simulink model "EV_motor_model"  (R2023a)
settings: Solver=ode15s  StartTime=0.0  StopTime=200  RelTol=1e-3
values from neighbouring files (symbols this model uses):
  A = 1.8    [evmodel.m]    (also in params.mat)
  B = 2e-4    (= 0.0002)    [evmodel.m]    (also in params.mat)
  Cd = 0.3    [evmodel.m]    (also in params.mat)
  G = 11    [params.mat]
  J = 0.05    [evmodel.m]    (also in params.mat)
  La = 0.003004    [params.mat]
  Laf = 0.001766    [evmodel.m]    (also in params.mat)
  Lf = 0.003004    [params.mat]
  m = 800    [evmodel.m]    (also in params.mat)
  mu_rr = 0.015    [params.mat]
  r = 0.25    [evmodel.m]    (also in params.mat = 0.3)
  Ra = 0.06    [params.mat]
  Rf = 0.06    [params.mat]
  rho = 1.25    [evmodel.m]    (also in params.mat)
undefined symbols (not defined in the file or in its folder): DiscIntNeverNeededParam
libraries: slpidlib x5, eePwmGenerator x1, spsTriangleGeneratorLib x1
settings Model: Creator=HP  LastModifiedBy=karti
settings DebuggingCC: AlgebraicLoopMsg=none  UnconnectedInputMsg=warning  UnconnectedOutputMsg=warning  UnconnectedLineMsg=warning
settings ModelReferenceCC: EnableRefExpFcnMdlSchedulingChecks=on
settings RTWCC: DLArmComputeVersion=19.05

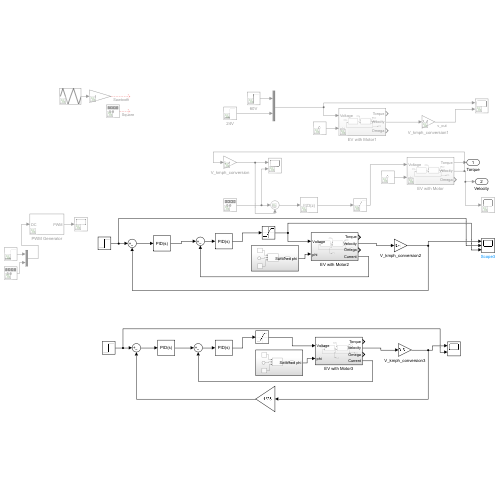
[thumbnail: Simulink's stored preview of the top-level diagram]
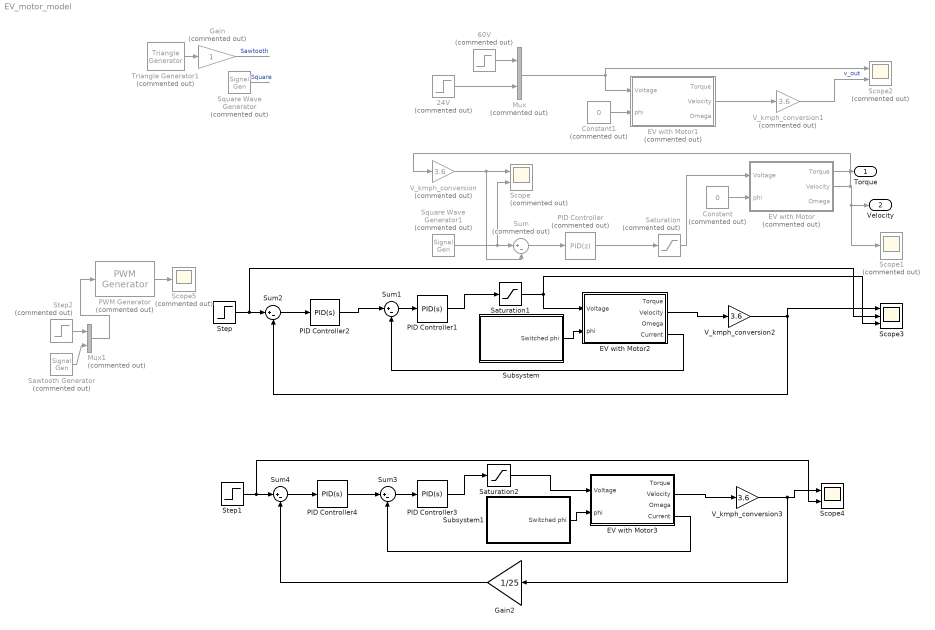
== system EV_motor_model ==
  24V : Step  Commented=on  Time=0  After=24  SampleTime=0
  60V : Step  Commented=on  Time=0  After=60  SampleTime=0
  Constant : Constant  Commented=on  Value=0
  Constant1 : Constant  Commented=on  Value=0
  EV with Motor : Subsystem  Commented=on
  EV with Motor1 : Subsystem  Commented=on
  EV with Motor2 : Subsystem
  EV with Motor3 : Subsystem
  Gain : Gain  Commented=on
  Gain2 : Gain  Gain=1/25
  Mux : Mux  Commented=on  Inputs=2
  Mux1 : Mux  Commented=on  Inputs=2
  PID Controller : slpidlib/PID Controller  Commented=on  Controller=PID  Form=Parallel  TimeDomain=Discrete-time  UseExternalTs=off  SampleTime=-1  IntegratorMethod=Forward Euler  FilterMethod=Forward Euler  ControllerParametersSource=internal  P=21.8052  I=4.7645  UseKiTs=off  D=2  N=100  UseFilter=on  TunerSelectOption=Frequency Response Based  InitialConditionSource=internal  InitialConditionForIntegrator=0  InitialConditionForFilter=0  DifferentiatorICPrevScaledInput=0  ExternalReset=none  TrackingMode=off  Kt=1  LimitOutput=off  SatLimitsSource=internal  UpperSaturationLimit=inf  LowerSaturationLimit=-inf  LinearizeAsGain=on  AntiWindupMode=none  Kb=1  LimitIntegrator=off  UpperIntegratorSaturationLimit=inf  LowerIntegratorSaturationLimit=-inf  POutMin=[]  POutMax=[]  IOutMin=[]  IOutMax=[]  DOutMin=[]  DOutMax=[]  NOutMin=[]  NOutMax=[]  SumOutMin=[]  SumOutMax=[]  SaturationOutMin=[]  SaturationOutMax=[]  PParamMin=[]  PParamMax=[]  IParamMin=[]  IParamMax=[]  DParamMin=[]  DParamMax=[]  NParamMin=[]  NParamMax=[]  KbParamMin=[]  KbParamMax=[]  KtParamMin=[]  KtParamMax=[]  KbOutMin=[]  KbOutMax=[]  KtOutMin=[]  KtOutMax=[]  IntegratorOutMin=[]  IntegratorOutMax=[]  FilterOutMin=[]  FilterOutMax=[]  SumI1OutMin=[]  SumI1OutMax=[]  SumI2OutMin=[]  SumI2OutMax=[]  SumI3OutMin=[]  SumI3OutMax=[]  SumI4OutMin=[]  SumI4OutMax=[]  SumDOutMin=[]  SumDOutMax=[]  DifferentiatorOutMin=[]  DifferentiatorOutMax=[]  FilterDiffOutCoefMin=[]  FilterDiffOutCoefMax=[]  ReciprocalOutMin=[]  ReciprocalOutMax=[]  SumDenOutMin=[]  SumDenOutMax=[]  SumNumOutMin=[]  SumNumOutMax=[]  DivideOutMin=[]  DivideOutMax=[]  UdiffTsProdOutMin=[]  UdiffTsProdOutMax=[]  NTsProdOutMin=[]  NTsProdOutMax=[]  UintegralTsProdOutMin=[]  UintegralTsProdOutMax=[]  UngainTsProdOutMin=[]  UngainTsProdOutMax=[]  ClampingZeroOutDataTypeStr=Inherit: Inherit via back propagation  ClampingZeroOutMin=[]  ClampingZeroOutMax=[]  FilterDenConstantOutDataTypeStr=Inherit: Inherit via back propagation  FilterDenConstantOutMin=[]  FilterDenConstantOutMax=[]  PCopyOutDataTypeStr=Inherit: Inherit via back propagation  PCopyOutMin=[]  PCopyOutMax=[]  NCopyOutDataTypeStr=Inherit: Inherit via back propagation  NCopyOutMin=[]  NCopyOutMax=[]  IntegratorContinuousStateAttributes=''  IntegratorStateMustResolveToSignalObject=off  IntegratorRTWStateStorageClass=Auto  FilterContinuousStateAttributes=''  FilterStateMustResolveToSignalObject=off  FilterRTWStateStorageClass=Auto  ParallelPVariant=InternalParameters  IdealPVariant=Disabled  IVariant=InternalParameters  DVariant=InternalParameters  IntegratorVariant=Discrete  SatVariant=Disabled  AWVariant=Passthrough  PCopyVariant=Disabled  TRVariant=Disabled  FdbkBlocksVariant=Forward  IdealPFdbkVariant=Disabled  SatFdbkVariant=Disabled  DerivativeFilterVariant=ForwardEulerFilter  NVariant=InternalParameters  NCopyVariant=Disabled  FilterICVariant=InternalICsFilter  IntegratorICVariant=InternalICs  ExternalResetVariant=Disabled  TRSumVariant=Passthrough  SumFdbkVariant=Disabled  SumVariant=Sum_PID  TsampFilterVariant=InternalTs  TsampNgainVariant=Passthrough  TsampIntegralVariant=Disabled_SignalSpec  ExternalSaturationOutDataTypeStr=Inherit: Same as second input
  PID Controller1 : slpidlib/PID Controller  Controller=PID  Form=Parallel  TimeDomain=Continuous-time  UseExternalTs=off  SampleTime=-1  IntegratorMethod=Forward Euler  FilterMethod=Forward Euler  ControllerParametersSource=internal  P=10.01  I=10.51  UseKiTs=off  D=100  N=100  UseFilter=on  TunerSelectOption=Frequency Response Based  InitialConditionSource=internal  InitialConditionForIntegrator=0  InitialConditionForFilter=0  DifferentiatorICPrevScaledInput=0  ExternalReset=none  TrackingMode=off  Kt=1  LimitOutput=off  SatLimitsSource=internal  UpperSaturationLimit=inf  LowerSaturationLimit=-inf  LinearizeAsGain=on  AntiWindupMode=none  Kb=1  LimitIntegrator=off  UpperIntegratorSaturationLimit=inf  LowerIntegratorSaturationLimit=-inf  POutMin=[]  POutMax=[]  IOutMin=[]  IOutMax=[]  DOutMin=[]  DOutMax=[]  NOutMin=[]  NOutMax=[]  SumOutMin=[]  SumOutMax=[]  SaturationOutMin=[]  SaturationOutMax=[]  PParamMin=[]  PParamMax=[]  IParamMin=[]  IParamMax=[]  DParamMin=[]  DParamMax=[]  NParamMin=[]  NParamMax=[]  KbParamMin=[]  KbParamMax=[]  KtParamMin=[]  KtParamMax=[]  KbOutMin=[]  KbOutMax=[]  KtOutMin=[]  KtOutMax=[]  IntegratorOutMin=[]  IntegratorOutMax=[]  FilterOutMin=[]  FilterOutMax=[]  SumI1OutMin=[]  SumI1OutMax=[]  SumI2OutMin=[]  SumI2OutMax=[]  SumI3OutMin=[]  SumI3OutMax=[]  SumI4OutMin=[]  SumI4OutMax=[]  SumDOutMin=[]  SumDOutMax=[]  DifferentiatorOutMin=[]  DifferentiatorOutMax=[]  FilterDiffOutCoefMin=[]  FilterDiffOutCoefMax=[]  ReciprocalOutMin=[]  ReciprocalOutMax=[]  SumDenOutMin=[]  SumDenOutMax=[]  SumNumOutMin=[]  SumNumOutMax=[]  DivideOutMin=[]  DivideOutMax=[]  UdiffTsProdOutMin=[]  UdiffTsProdOutMax=[]  NTsProdOutMin=[]  NTsProdOutMax=[]  UintegralTsProdOutMin=[]  UintegralTsProdOutMax=[]  UngainTsProdOutMin=[]  UngainTsProdOutMax=[]  ClampingZeroOutDataTypeStr=Inherit: Inherit via back propagation  ClampingZeroOutMin=[]  ClampingZeroOutMax=[]  FilterDenConstantOutDataTypeStr=Inherit: Inherit via back propagation  FilterDenConstantOutMin=[]  FilterDenConstantOutMax=[]  PCopyOutDataTypeStr=Inherit: Inherit via back propagation  PCopyOutMin=[]  PCopyOutMax=[]  NCopyOutDataTypeStr=Inherit: Inherit via back propagation  NCopyOutMin=[]  NCopyOutMax=[]  IntegratorContinuousStateAttributes=''  IntegratorStateMustResolveToSignalObject=off  IntegratorRTWStateStorageClass=Auto  FilterContinuousStateAttributes=''  FilterStateMustResolveToSignalObject=off  FilterRTWStateStorageClass=Auto  ParallelPVariant=InternalParameters  IdealPVariant=Disabled  IVariant=InternalParameters  DVariant=InternalParameters  IntegratorVariant=Continuous  SatVariant=Disabled  AWVariant=Passthrough  PCopyVariant=Disabled  TRVariant=Disabled  FdbkBlocksVariant=Forward  IdealPFdbkVariant=Disabled  SatFdbkVariant=Disabled  DerivativeFilterVariant=ContFilter  NVariant=InternalParameters  NCopyVariant=Disabled  FilterICVariant=InternalICsFilter  IntegratorICVariant=InternalICs  ExternalResetVariant=Disabled  TRSumVariant=Passthrough  SumFdbkVariant=Disabled  SumVariant=Sum_PID  TsampFilterVariant=InternalTs  TsampNgainVariant=Passthrough  TsampIntegralVariant=Disabled_SignalSpec  ExternalSaturationOutDataTypeStr=Inherit: Same as second input
  PID Controller2 : slpidlib/PID Controller  Controller=PID  Form=Parallel  TimeDomain=Continuous-time  UseExternalTs=off  SampleTime=-1  IntegratorMethod=Forward Euler  FilterMethod=Forward Euler  ControllerParametersSource=internal  P=10.01  I=10.01  UseKiTs=off  D=0.1  N=100  UseFilter=on  TunerSelectOption=Frequency Response Based  InitialConditionSource=internal  InitialConditionForIntegrator=0  InitialConditionForFilter=0  DifferentiatorICPrevScaledInput=0  ExternalReset=none  TrackingMode=off  Kt=1  LimitOutput=off  SatLimitsSource=internal  UpperSaturationLimit=inf  LowerSaturationLimit=-inf  LinearizeAsGain=on  AntiWindupMode=none  Kb=1  LimitIntegrator=off  UpperIntegratorSaturationLimit=inf  LowerIntegratorSaturationLimit=-inf  POutMin=[]  POutMax=[]  IOutMin=[]  IOutMax=[]  DOutMin=[]  DOutMax=[]  NOutMin=[]  NOutMax=[]  SumOutMin=[]  SumOutMax=[]  SaturationOutMin=[]  SaturationOutMax=[]  PParamMin=[]  PParamMax=[]  IParamMin=[]  IParamMax=[]  DParamMin=[]  DParamMax=[]  NParamMin=[]  NParamMax=[]  KbParamMin=[]  KbParamMax=[]  KtParamMin=[]  KtParamMax=[]  KbOutMin=[]  KbOutMax=[]  KtOutMin=[]  KtOutMax=[]  IntegratorOutMin=[]  IntegratorOutMax=[]  FilterOutMin=[]  FilterOutMax=[]  SumI1OutMin=[]  SumI1OutMax=[]  SumI2OutMin=[]  SumI2OutMax=[]  SumI3OutMin=[]  SumI3OutMax=[]  SumI4OutMin=[]  SumI4OutMax=[]  SumDOutMin=[]  SumDOutMax=[]  DifferentiatorOutMin=[]  DifferentiatorOutMax=[]  FilterDiffOutCoefMin=[]  FilterDiffOutCoefMax=[]  ReciprocalOutMin=[]  ReciprocalOutMax=[]  SumDenOutMin=[]  SumDenOutMax=[]  SumNumOutMin=[]  SumNumOutMax=[]  DivideOutMin=[]  DivideOutMax=[]  UdiffTsProdOutMin=[]  UdiffTsProdOutMax=[]  NTsProdOutMin=[]  NTsProdOutMax=[]  UintegralTsProdOutMin=[]  UintegralTsProdOutMax=[]  UngainTsProdOutMin=[]  UngainTsProdOutMax=[]  ClampingZeroOutDataTypeStr=Inherit: Inherit via back propagation  ClampingZeroOutMin=[]  ClampingZeroOutMax=[]  FilterDenConstantOutDataTypeStr=Inherit: Inherit via back propagation  FilterDenConstantOutMin=[]  FilterDenConstantOutMax=[]  PCopyOutDataTypeStr=Inherit: Inherit via back propagation  PCopyOutMin=[]  PCopyOutMax=[]  NCopyOutDataTypeStr=Inherit: Inherit via back propagation  NCopyOutMin=[]  NCopyOutMax=[]  IntegratorContinuousStateAttributes=''  IntegratorStateMustResolveToSignalObject=off  IntegratorRTWStateStorageClass=Auto  FilterContinuousStateAttributes=''  FilterStateMustResolveToSignalObject=off  FilterRTWStateStorageClass=Auto  ParallelPVariant=InternalParameters  IdealPVariant=Disabled  IVariant=InternalParameters  DVariant=InternalParameters  IntegratorVariant=Continuous  SatVariant=Disabled  AWVariant=Passthrough  PCopyVariant=Disabled  TRVariant=Disabled  FdbkBlocksVariant=Forward  IdealPFdbkVariant=Disabled  SatFdbkVariant=Disabled  DerivativeFilterVariant=ContFilter  NVariant=InternalParameters  NCopyVariant=Disabled  FilterICVariant=InternalICsFilter  IntegratorICVariant=InternalICs  ExternalResetVariant=Disabled  TRSumVariant=Passthrough  SumFdbkVariant=Disabled  SumVariant=Sum_PID  TsampFilterVariant=InternalTs  TsampNgainVariant=Passthrough  TsampIntegralVariant=Disabled_SignalSpec  ExternalSaturationOutDataTypeStr=Inherit: Same as second input
  PID Controller3 : slpidlib/PID Controller  Controller=PID  Form=Parallel  TimeDomain=Continuous-time  UseExternalTs=off  SampleTime=-1  IntegratorMethod=Forward Euler  FilterMethod=Forward Euler  ControllerParametersSource=internal  P=0.1  I=2  UseKiTs=off  D=0  N=100  UseFilter=on  TunerSelectOption=Frequency Response Based  InitialConditionSource=internal  InitialConditionForIntegrator=0  InitialConditionForFilter=0  DifferentiatorICPrevScaledInput=0  ExternalReset=none  TrackingMode=off  Kt=1  LimitOutput=off  SatLimitsSource=internal  UpperSaturationLimit=inf  LowerSaturationLimit=-inf  LinearizeAsGain=on  AntiWindupMode=none  Kb=1  LimitIntegrator=off  UpperIntegratorSaturationLimit=inf  LowerIntegratorSaturationLimit=-inf  POutMin=[]  POutMax=[]  IOutMin=[]  IOutMax=[]  DOutMin=[]  DOutMax=[]  NOutMin=[]  NOutMax=[]  SumOutMin=[]  SumOutMax=[]  SaturationOutMin=[]  SaturationOutMax=[]  PParamMin=[]  PParamMax=[]  IParamMin=[]  IParamMax=[]  DParamMin=[]  DParamMax=[]  NParamMin=[]  NParamMax=[]  KbParamMin=[]  KbParamMax=[]  KtParamMin=[]  KtParamMax=[]  KbOutMin=[]  KbOutMax=[]  KtOutMin=[]  KtOutMax=[]  IntegratorOutMin=[]  IntegratorOutMax=[]  FilterOutMin=[]  FilterOutMax=[]  SumI1OutMin=[]  SumI1OutMax=[]  SumI2OutMin=[]  SumI2OutMax=[]  SumI3OutMin=[]  SumI3OutMax=[]  SumI4OutMin=[]  SumI4OutMax=[]  SumDOutMin=[]  SumDOutMax=[]  DifferentiatorOutMin=[]  DifferentiatorOutMax=[]  FilterDiffOutCoefMin=[]  FilterDiffOutCoefMax=[]  ReciprocalOutMin=[]  ReciprocalOutMax=[]  SumDenOutMin=[]  SumDenOutMax=[]  SumNumOutMin=[]  SumNumOutMax=[]  DivideOutMin=[]  DivideOutMax=[]  UdiffTsProdOutMin=[]  UdiffTsProdOutMax=[]  NTsProdOutMin=[]  NTsProdOutMax=[]  UintegralTsProdOutMin=[]  UintegralTsProdOutMax=[]  UngainTsProdOutMin=[]  UngainTsProdOutMax=[]  ClampingZeroOutDataTypeStr=Inherit: Inherit via back propagation  ClampingZeroOutMin=[]  ClampingZeroOutMax=[]  FilterDenConstantOutDataTypeStr=Inherit: Inherit via back propagation  FilterDenConstantOutMin=[]  FilterDenConstantOutMax=[]  PCopyOutDataTypeStr=Inherit: Inherit via back propagation  PCopyOutMin=[]  PCopyOutMax=[]  NCopyOutDataTypeStr=Inherit: Inherit via back propagation  NCopyOutMin=[]  NCopyOutMax=[]  IntegratorContinuousStateAttributes=''  IntegratorStateMustResolveToSignalObject=off  IntegratorRTWStateStorageClass=Auto  FilterContinuousStateAttributes=''  FilterStateMustResolveToSignalObject=off  FilterRTWStateStorageClass=Auto  ParallelPVariant=InternalParameters  IdealPVariant=Disabled  IVariant=InternalParameters  DVariant=InternalParameters  IntegratorVariant=Continuous  SatVariant=Disabled  AWVariant=Passthrough  PCopyVariant=Disabled  TRVariant=Disabled  FdbkBlocksVariant=Forward  IdealPFdbkVariant=Disabled  SatFdbkVariant=Disabled  DerivativeFilterVariant=ContFilter  NVariant=InternalParameters  NCopyVariant=Disabled  FilterICVariant=InternalICsFilter  IntegratorICVariant=InternalICs  ExternalResetVariant=Disabled  TRSumVariant=Passthrough  SumFdbkVariant=Disabled  SumVariant=Sum_PID  TsampFilterVariant=InternalTs  TsampNgainVariant=Passthrough  TsampIntegralVariant=Disabled_SignalSpec  ExternalSaturationOutDataTypeStr=Inherit: Same as second input
  PID Controller4 : slpidlib/PID Controller  Controller=PID  Form=Parallel  TimeDomain=Continuous-time  UseExternalTs=off  SampleTime=-1  IntegratorMethod=Forward Euler  FilterMethod=Forward Euler  ControllerParametersSource=internal  P=150  I=20  UseKiTs=off  D=1  N=100  UseFilter=on  TunerSelectOption=Frequency Response Based  InitialConditionSource=internal  InitialConditionForIntegrator=0  InitialConditionForFilter=0  DifferentiatorICPrevScaledInput=0  ExternalReset=none  TrackingMode=off  Kt=1  LimitOutput=off  SatLimitsSource=internal  UpperSaturationLimit=inf  LowerSaturationLimit=-inf  LinearizeAsGain=on  AntiWindupMode=none  Kb=1  LimitIntegrator=off  UpperIntegratorSaturationLimit=inf  LowerIntegratorSaturationLimit=-inf  POutMin=[]  POutMax=[]  IOutMin=[]  IOutMax=[]  DOutMin=[]  DOutMax=[]  NOutMin=[]  NOutMax=[]  SumOutMin=[]  SumOutMax=[]  SaturationOutMin=[]  SaturationOutMax=[]  PParamMin=[]  PParamMax=[]  IParamMin=[]  IParamMax=[]  DParamMin=[]  DParamMax=[]  NParamMin=[]  NParamMax=[]  KbParamMin=[]  KbParamMax=[]  KtParamMin=[]  KtParamMax=[]  KbOutMin=[]  KbOutMax=[]  KtOutMin=[]  KtOutMax=[]  IntegratorOutMin=[]  IntegratorOutMax=[]  FilterOutMin=[]  FilterOutMax=[]  SumI1OutMin=[]  SumI1OutMax=[]  SumI2OutMin=[]  SumI2OutMax=[]  SumI3OutMin=[]  SumI3OutMax=[]  SumI4OutMin=[]  SumI4OutMax=[]  SumDOutMin=[]  SumDOutMax=[]  DifferentiatorOutMin=[]  DifferentiatorOutMax=[]  FilterDiffOutCoefMin=[]  FilterDiffOutCoefMax=[]  ReciprocalOutMin=[]  ReciprocalOutMax=[]  SumDenOutMin=[]  SumDenOutMax=[]  SumNumOutMin=[]  SumNumOutMax=[]  DivideOutMin=[]  DivideOutMax=[]  UdiffTsProdOutMin=[]  UdiffTsProdOutMax=[]  NTsProdOutMin=[]  NTsProdOutMax=[]  UintegralTsProdOutMin=[]  UintegralTsProdOutMax=[]  UngainTsProdOutMin=[]  UngainTsProdOutMax=[]  ClampingZeroOutDataTypeStr=Inherit: Inherit via back propagation  ClampingZeroOutMin=[]  ClampingZeroOutMax=[]  FilterDenConstantOutDataTypeStr=Inherit: Inherit via back propagation  FilterDenConstantOutMin=[]  FilterDenConstantOutMax=[]  PCopyOutDataTypeStr=Inherit: Inherit via back propagation  PCopyOutMin=[]  PCopyOutMax=[]  NCopyOutDataTypeStr=Inherit: Inherit via back propagation  NCopyOutMin=[]  NCopyOutMax=[]  IntegratorContinuousStateAttributes=''  IntegratorStateMustResolveToSignalObject=off  IntegratorRTWStateStorageClass=Auto  FilterContinuousStateAttributes=''  FilterStateMustResolveToSignalObject=off  FilterRTWStateStorageClass=Auto  ParallelPVariant=InternalParameters  IdealPVariant=Disabled  IVariant=InternalParameters  DVariant=InternalParameters  IntegratorVariant=Continuous  SatVariant=Disabled  AWVariant=Passthrough  PCopyVariant=Disabled  TRVariant=Disabled  FdbkBlocksVariant=Forward  IdealPFdbkVariant=Disabled  SatFdbkVariant=Disabled  DerivativeFilterVariant=ContFilter  NVariant=InternalParameters  NCopyVariant=Disabled  FilterICVariant=InternalICsFilter  IntegratorICVariant=InternalICs  ExternalResetVariant=Disabled  TRSumVariant=Passthrough  SumFdbkVariant=Disabled  SumVariant=Sum_PID  TsampFilterVariant=InternalTs  TsampNgainVariant=Passthrough  TsampIntegralVariant=Disabled_SignalSpec  ExternalSaturationOutDataTypeStr=Inherit: Same as second input
  PWM Generator : eePwmGenerator/PWM Generator  Commented=on  CarrCount=Up  Tper=0.1  Tdelay=0  Ts=5e-5
  Saturation : Saturate  Commented=on  UpperLimit=25  LowerLimit=-25
  Saturation1 : Saturate  UpperLimit=48  LowerLimit=-48
  Saturation2 : Saturate  UpperLimit=48  LowerLimit=-48
  Sawtooth Generator : SignalGenerator  Commented=on  WaveForm=sawtooth  Units=rad/sec
  Scope : Scope  Commented=on  NumInputPorts=2
  Scope1 : Scope  Commented=on
  Scope2 : Scope  Commented=on  NumInputPorts=2
  Scope3 : Scope  NumInputPorts=3
  Scope4 : Scope  NumInputPorts=2
  Scope5 : Scope  Commented=on
  Square Wave Generator : SignalGenerator  Commented=on  WaveForm=square  Amplitude=20  Frequency=1/20
  Square Wave Generator1 : SignalGenerator  Commented=on  WaveForm=square  Amplitude=20  Frequency=1/20
  Step : Step  After=10  SampleTime=0
  Step1 : Step  After=10  SampleTime=0
  Step2 : Step  Commented=on  After=30  SampleTime=0
  Subsystem : Subsystem
  Subsystem1 : Subsystem
  Sum : Sum  Commented=on  Inputs=|+-
  Sum{1..4} (4 alike) : Sum  Inputs=|+-
  Triangle Generator1 : spsTriangleGeneratorLib/Triangle Generator  Commented=on  Freq=1/20  Phase=90  Ts=0
  V_kmph_conversion : Gain  Commented=on  Gain=3.6
  V_kmph_conversion1 : Gain  Commented=on  Gain=3.6
  V_kmph_conversion2 : Gain  Gain=3.6
  V_kmph_conversion3 : Gain  Gain=3.6
  Torque : Outport
  Velocity : Outport  Port=2
  wires:
  60V/1 -> Mux/1
  24V/1 -> Mux/2
  V_kmph_conversion/1 -> Sum/2, Scope/1
  Square Wave Generator1/1 -> Sum/1, Scope/2
  Sum/1 -> PID Controller/1
  Mux/1 -> EV with Motor1/1(Voltage), Scope2/1
  Constant1/1 -> EV with Motor1/2(phi)
  PID Controller/1 -> Saturation/1
  EV with Motor/1(Torque) -> Torque/1
  EV with Motor1/2(Velocity) -> V_kmph_conversion1/1
  Constant/1 -> EV with Motor/2(phi)
  Saturation/1 -> EV with Motor/1(Voltage)
  V_kmph_conversion1/1 -> Scope2/2  "v_out"
  EV with Motor/2(Velocity) -> V_kmph_conversion/1, Scope1/1, Velocity/1
  Saturation1/1 -> EV with Motor2/1(Voltage), Scope3/3
  PID Controller1/1 -> Saturation1/1
  Sum2/1 -> PID Controller2/1
  PID Controller2/1 -> Sum1/1
  Sum1/1 -> PID Controller1/1
  V_kmph_conversion2/1 -> Sum2/2, Scope3/1
  EV with Motor2/4(Current) -> Sum1/2
  Step/1 -> Sum2/1, Scope3/2
  Subsystem/1(Switched phi) -> EV with Motor2/2(phi)
  EV with Motor3/4(Current) -> Sum3/2
  Step1/1 -> Sum4/1, Scope4/2
  Subsystem1/1(Switched phi) -> EV with Motor3/2(phi)
  Gain2/1 -> Sum4/2
  V_kmph_conversion3/1 -> Gain2/1, Scope4/1
  EV with Motor3/2(Velocity) -> V_kmph_conversion3/1
  Sum3/1 -> PID Controller3/1
  PID Controller4/1 -> Sum3/1
  Sum4/1 -> PID Controller4/1
  Saturation2/1 -> EV with Motor3/1(Voltage)
  PID Controller3/1 -> Saturation2/1
  EV with Motor2/2(Velocity) -> V_kmph_conversion2/1
  Gain/1 -> ?  "Sawtooth"
  Triangle Generator1/1 -> Gain/1
  Square Wave Generator/1 -> ?  "Square"
  PWM Generator/1 -> Scope5/1
  Step2/1 -> Mux1/1
  Mux1/1 -> PWM Generator/1
  Sawtooth Generator/1 -> Mux1/2

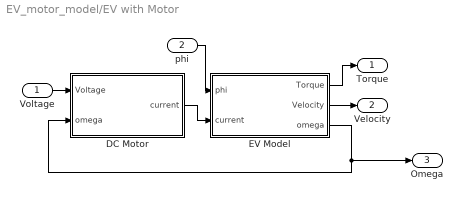
== system EV_motor_model/EV with Motor ==
  Voltage : Inport
  phi : Inport  Port=2
  DC Motor : Subsystem
  EV Model : Subsystem
  Torque : Outport
  Velocity : Outport  Port=2
  Omega : Outport  Port=3
  wires:
  EV Model/1(Torque) -> Torque/1
  DC Motor/1(current) -> EV Model/2(current)
  phi/1 -> EV Model/1(phi)
  EV Model/3(omega) -> Omega/1, DC Motor/2(omega)
  Voltage/1 -> DC Motor/1(Voltage)
  EV Model/2(Velocity) -> Velocity/1

== system EV_motor_model/EV with Motor1 ==
  Voltage : Inport
  phi : Inport  Port=2
  DC Motor : Subsystem
  EV Model : Subsystem
  Torque : Outport
  Velocity : Outport  Port=2
  Omega : Outport  Port=3
  wires:
  EV Model/1(Torque) -> Torque/1
  DC Motor/1(current) -> EV Model/2(current)
  phi/1 -> EV Model/1(phi)
  EV Model/3(omega) -> Omega/1, DC Motor/2(omega)
  Voltage/1 -> DC Motor/1(Voltage)
  EV Model/2(Velocity) -> Velocity/1

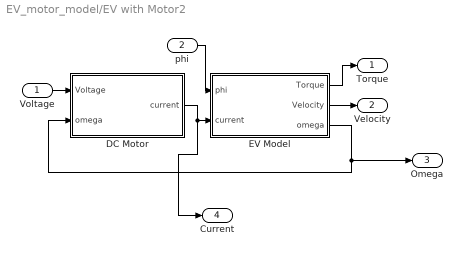
== system EV_motor_model/EV with Motor2 ==
  Voltage : Inport
  phi : Inport  Port=2
  DC Motor : Subsystem
  EV Model : Subsystem
  Torque : Outport
  Velocity : Outport  Port=2
  Omega : Outport  Port=3
  Current : Outport  Port=4
  wires:
  EV Model/1(Torque) -> Torque/1
  DC Motor/1(current) -> Current/1, EV Model/2(current)
  phi/1 -> EV Model/1(phi)
  EV Model/3(omega) -> Omega/1, DC Motor/2(omega)
  Voltage/1 -> DC Motor/1(Voltage)
  EV Model/2(Velocity) -> Velocity/1

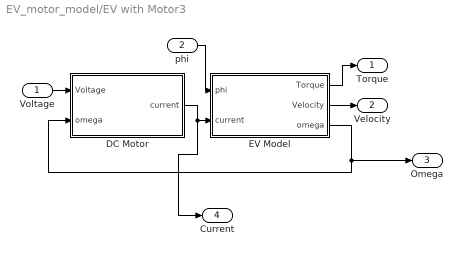
== system EV_motor_model/EV with Motor3 ==
  Voltage : Inport
  phi : Inport  Port=2
  DC Motor : Subsystem
  EV Model : Subsystem
  Torque : Outport
  Velocity : Outport  Port=2
  Omega : Outport  Port=3
  Current : Outport  Port=4
  wires:
  EV Model/1(Torque) -> Torque/1
  DC Motor/1(current) -> Current/1, EV Model/2(current)
  phi/1 -> EV Model/1(phi)
  EV Model/3(omega) -> Omega/1, DC Motor/2(omega)
  Voltage/1 -> DC Motor/1(Voltage)
  EV Model/2(Velocity) -> Velocity/1

== system EV_motor_model/Subsystem ==
  Clock : Clock
  Constant2 : Constant  Value=0
  Constant3 : Constant  Value=0.01
  Switch : Switch  Threshold=10  SaturateOnIntegerOverflow=off  InputSameDT=off
  Switched phi : Outport
  wires:
  Constant2/1 -> Switch/3
  Constant3/1 -> Switch/1
  Clock/1 -> Switch/2
  Switch/1 -> Switched phi/1

== system EV_motor_model/Subsystem1 ==
  Clock : Clock
  Constant2 : Constant  Value=0
  Constant3 : Constant  Value=0.01
  Switch : Switch  Threshold=10  SaturateOnIntegerOverflow=off  InputSameDT=off
  Switched phi : Outport
  wires:
  Constant2/1 -> Switch/3
  Constant3/1 -> Switch/1
  Clock/1 -> Switch/2
  Switch/1 -> Switched phi/1

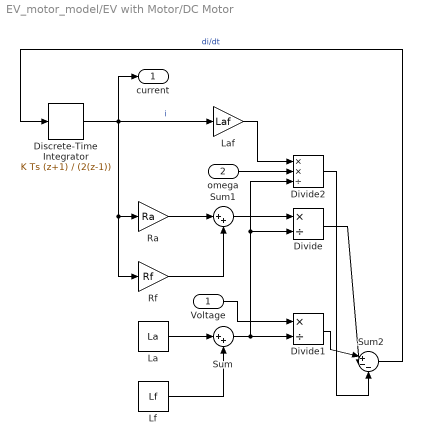
== system EV_motor_model/EV with Motor/DC Motor ==
  Voltage : Inport
  omega : Inport  Port=2
  Discrete-Time Integrator : DiscreteIntegrator  IntegratorMethod=Integration: Trapezoidal  SampleTime=-1  ICPrevOutput=DiscIntNeverNeededParam  ICPrevScaledInput=DiscIntNeverNeededParam
  Divide : Product  Inputs=*/
  Divide1 : Product  Inputs=*/
  Divide2 : Product  Inputs=**/
  La : Constant  Value=La
  Laf : Gain  Gain=Laf
  Lf : Constant  Value=Lf
  Ra : Gain  Gain=Ra
  Rf : Gain  Gain=Rf
  Sum : Sum  Inputs=|++
  Sum1 : Sum  Inputs=|++
  Sum2 : Sum  Inputs=|+--
  current : Outport
  wires:
  La/1 -> Sum/1
  Divide2/1 -> Sum2/3
  Lf/1 -> Sum/2
  Discrete-Time Integrator/1 -> Rf/1, Ra/1, current/1, Laf/1  "i"
  Ra/1 -> Sum1/1
  Rf/1 -> Sum1/2
  omega/1 -> Divide2/2
  Divide1/1 -> Sum2/1
  Sum/1 -> Divide2/3, Divide/2, Divide1/2
  Voltage/1 -> Divide1/1
  Laf/1 -> Divide2/1
  Divide/1 -> Sum2/2
  Sum1/1 -> Divide/1
  Sum2/1 -> Discrete-Time Integrator/1  "di/dt"

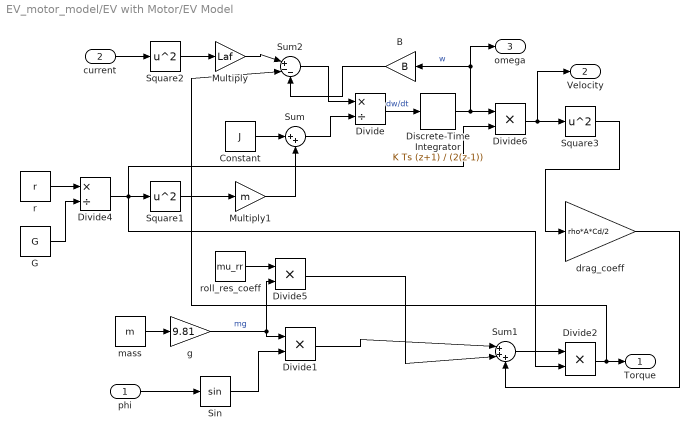
== system EV_motor_model/EV with Motor/EV Model ==
  phi : Inport
  current : Inport  Port=2
  B : Gain  Gain=B
  Constant : Constant  Value=J
  Discrete-Time Integrator : DiscreteIntegrator  IntegratorMethod=Integration: Trapezoidal  SampleTime=-1  ICPrevOutput=DiscIntNeverNeededParam  ICPrevScaledInput=DiscIntNeverNeededParam
  Divide : Product  Inputs=*/
  Divide{1..2,5..6} (4 alike) : Product  Inputs=**
  Divide4 : Product  Inputs=*/
  G : Constant  Value=G
  Multiply : Gain  Gain=Laf
  Multiply1 : Gain  Gain=m
  Sin : Trigonometry
  Square1 : Math  Operator=square
  Square2 : Math  Operator=square
  Square3 : Math  Operator=square
  Sum : Sum  Inputs=|++
  Sum1 : Sum  Inputs=|+++
  Sum2 : Sum  Inputs=|+--
  drag_coeff : Gain  Gain=rho*A*Cd/2
  g : Gain  Gain=9.81
  mass : Constant  Value=m
  r : Constant  Value=r
  roll_res_coeff : Constant  Value=mu_rr
  Torque : Outport
  Velocity : Outport  Port=2
  omega : Outport  Port=3
  wires:
  Sum/1 -> Divide/2
  Divide6/1 -> Velocity/1, Square3/1
  g/1 -> Divide5/2, Divide1/1  "mg"
  current/1 -> Square2/1
  B/1 -> Sum2/3
  Constant/1 -> Sum/1
  Multiply1/1 -> Sum/2
  r/1 -> Divide4/1
  Sum1/1 -> Divide2/1
  Square1/1 -> Multiply1/1
  Sum2/1 -> Divide/1
  Discrete-Time Integrator/1 -> Divide6/1, omega/1, B/1  "w"
  phi/1 -> Sin/1
  roll_res_coeff/1 -> Divide5/1
  Multiply/1 -> Sum2/1
  Divide1/1 -> Sum1/1
  Square2/1 -> Multiply/1
  Divide5/1 -> Sum1/2
  mass/1 -> g/1
  Square3/1 -> drag_coeff/1
  G/1 -> Divide4/2
  Divide4/1 -> Divide6/2, Divide2/2, Square1/1
  drag_coeff/1 -> Sum1/3
  Divide2/1 -> Sum2/2, Torque/1
  Sin/1 -> Divide1/2
  Divide/1 -> Discrete-Time Integrator/1  "dw/dt"

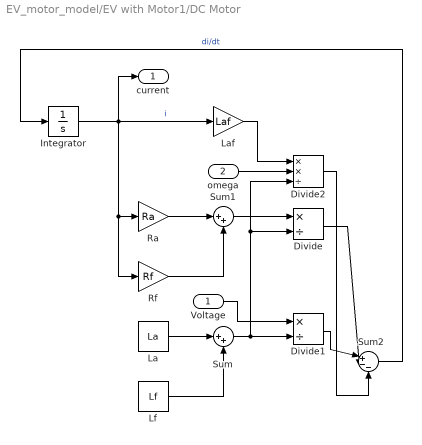
== system EV_motor_model/EV with Motor1/DC Motor ==
  Voltage : Inport
  omega : Inport  Port=2
  Divide : Product  Inputs=*/
  Divide1 : Product  Inputs=*/
  Divide2 : Product  Inputs=**/
  Integrator : Integrator
  La : Constant  Value=La
  Laf : Gain  Gain=Laf
  Lf : Constant  Value=Lf
  Ra : Gain  Gain=Ra
  Rf : Gain  Gain=Rf
  Sum : Sum  Inputs=|++
  Sum1 : Sum  Inputs=|++
  Sum2 : Sum  Inputs=|+--
  current : Outport
  wires:
  La/1 -> Sum/1
  Divide2/1 -> Sum2/3
  Lf/1 -> Sum/2
  Integrator/1 -> Rf/1, Ra/1, current/1, Laf/1  "i"
  Ra/1 -> Sum1/1
  Rf/1 -> Sum1/2
  omega/1 -> Divide2/2
  Divide1/1 -> Sum2/1
  Sum/1 -> Divide2/3, Divide/2, Divide1/2
  Voltage/1 -> Divide1/1
  Laf/1 -> Divide2/1
  Divide/1 -> Sum2/2
  Sum1/1 -> Divide/1
  Sum2/1 -> Integrator/1  "di/dt"

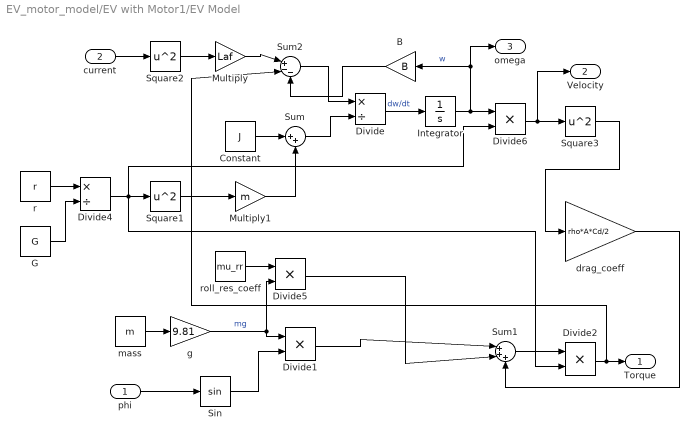
== system EV_motor_model/EV with Motor1/EV Model ==
  phi : Inport
  current : Inport  Port=2
  B : Gain  Gain=B
  Constant : Constant  Value=J
  Divide : Product  Inputs=*/
  Divide{1..2,5..6} (4 alike) : Product  Inputs=**
  Divide4 : Product  Inputs=*/
  G : Constant  Value=G
  Integrator : Integrator
  Multiply : Gain  Gain=Laf
  Multiply1 : Gain  Gain=m
  Sin : Trigonometry
  Square1 : Math  Operator=square
  Square2 : Math  Operator=square
  Square3 : Math  Operator=square
  Sum : Sum  Inputs=|++
  Sum1 : Sum  Inputs=|+++
  Sum2 : Sum  Inputs=|+--
  drag_coeff : Gain  Gain=rho*A*Cd/2
  g : Gain  Gain=9.81
  mass : Constant  Value=m
  r : Constant  Value=r
  roll_res_coeff : Constant  Value=mu_rr
  Torque : Outport
  Velocity : Outport  Port=2
  omega : Outport  Port=3
  wires:
  Sum/1 -> Divide/2
  Divide6/1 -> Velocity/1, Square3/1
  g/1 -> Divide5/2, Divide1/1  "mg"
  current/1 -> Square2/1
  B/1 -> Sum2/3
  Constant/1 -> Sum/1
  Multiply1/1 -> Sum/2
  r/1 -> Divide4/1
  Sum1/1 -> Divide2/1
  Square1/1 -> Multiply1/1
  Sum2/1 -> Divide/1
  Integrator/1 -> Divide6/1, omega/1, B/1  "w"
  phi/1 -> Sin/1
  roll_res_coeff/1 -> Divide5/1
  Multiply/1 -> Sum2/1
  Divide1/1 -> Sum1/1
  Square2/1 -> Multiply/1
  Divide5/1 -> Sum1/2
  mass/1 -> g/1
  Square3/1 -> drag_coeff/1
  G/1 -> Divide4/2
  Divide/1 -> Integrator/1  "dw/dt"
  Divide4/1 -> Divide6/2, Divide2/2, Square1/1
  drag_coeff/1 -> Sum1/3
  Divide2/1 -> Sum2/2, Torque/1
  Sin/1 -> Divide1/2

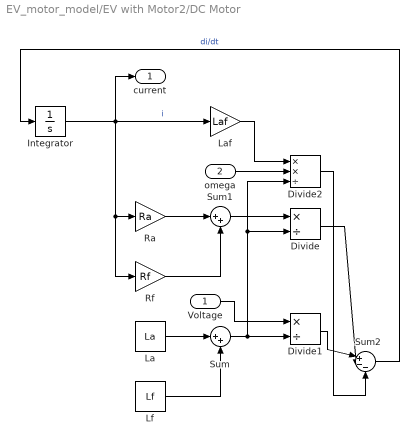
== system EV_motor_model/EV with Motor2/DC Motor ==
  Voltage : Inport
  omega : Inport  Port=2
  Divide : Product  Inputs=*/
  Divide1 : Product  Inputs=*/
  Divide2 : Product  Inputs=**/
  Integrator : Integrator
  La : Constant  Value=La
  Laf : Gain  Gain=Laf
  Lf : Constant  Value=Lf
  Ra : Gain  Gain=Ra
  Rf : Gain  Gain=Rf
  Sum : Sum  Inputs=|++
  Sum1 : Sum  Inputs=|++
  Sum2 : Sum  Inputs=|+--
  current : Outport
  wires:
  La/1 -> Sum/1
  Divide2/1 -> Sum2/3
  Lf/1 -> Sum/2
  Integrator/1 -> Rf/1, Ra/1, current/1, Laf/1  "i"
  Ra/1 -> Sum1/1
  Rf/1 -> Sum1/2
  omega/1 -> Divide2/2
  Divide1/1 -> Sum2/1
  Sum/1 -> Divide2/3, Divide/2, Divide1/2
  Voltage/1 -> Divide1/1
  Laf/1 -> Divide2/1
  Divide/1 -> Sum2/2
  Sum1/1 -> Divide/1
  Sum2/1 -> Integrator/1  "di/dt"

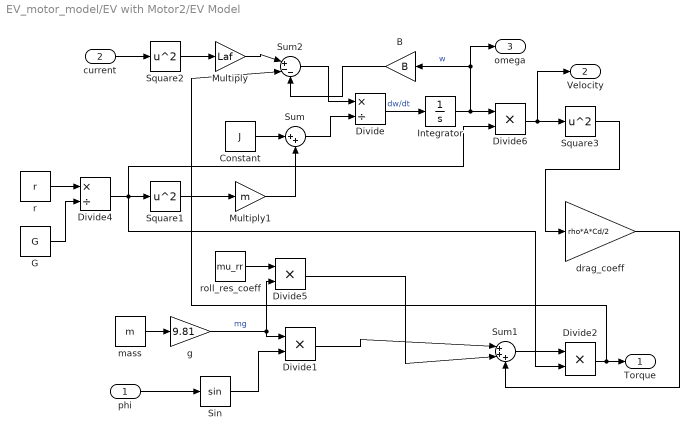
== system EV_motor_model/EV with Motor2/EV Model ==
  phi : Inport
  current : Inport  Port=2
  B : Gain  Gain=B
  Constant : Constant  Value=J
  Divide : Product  Inputs=*/
  Divide{1..2,5..6} (4 alike) : Product  Inputs=**
  Divide4 : Product  Inputs=*/
  G : Constant  Value=G
  Integrator : Integrator
  Multiply : Gain  Gain=Laf
  Multiply1 : Gain  Gain=m
  Sin : Trigonometry
  Square1 : Math  Operator=square
  Square2 : Math  Operator=square
  Square3 : Math  Operator=square
  Sum : Sum  Inputs=|++
  Sum1 : Sum  Inputs=|+++
  Sum2 : Sum  Inputs=|+--
  drag_coeff : Gain  Gain=rho*A*Cd/2
  g : Gain  Gain=9.81
  mass : Constant  Value=m
  r : Constant  Value=r
  roll_res_coeff : Constant  Value=mu_rr
  Torque : Outport
  Velocity : Outport  Port=2
  omega : Outport  Port=3
  wires:
  Sum/1 -> Divide/2
  Divide6/1 -> Velocity/1, Square3/1
  g/1 -> Divide5/2, Divide1/1  "mg"
  current/1 -> Square2/1
  B/1 -> Sum2/3
  Constant/1 -> Sum/1
  Multiply1/1 -> Sum/2
  r/1 -> Divide4/1
  Sum1/1 -> Divide2/1
  Square1/1 -> Multiply1/1
  Sum2/1 -> Divide/1
  Integrator/1 -> Divide6/1, omega/1, B/1  "w"
  phi/1 -> Sin/1
  roll_res_coeff/1 -> Divide5/1
  Multiply/1 -> Sum2/1
  Divide1/1 -> Sum1/1
  Square2/1 -> Multiply/1
  Divide5/1 -> Sum1/2
  mass/1 -> g/1
  Square3/1 -> drag_coeff/1
  G/1 -> Divide4/2
  Divide/1 -> Integrator/1  "dw/dt"
  Divide4/1 -> Divide6/2, Divide2/2, Square1/1
  drag_coeff/1 -> Sum1/3
  Divide2/1 -> Sum2/2, Torque/1
  Sin/1 -> Divide1/2

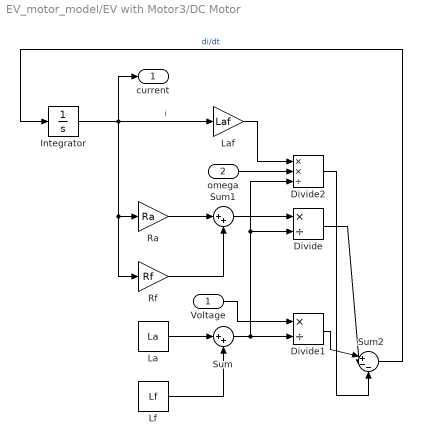
== system EV_motor_model/EV with Motor3/DC Motor ==
  Voltage : Inport
  omega : Inport  Port=2
  Divide : Product  Inputs=*/
  Divide1 : Product  Inputs=*/
  Divide2 : Product  Inputs=**/
  Integrator : Integrator
  La : Constant  Value=La
  Laf : Gain  Gain=Laf
  Lf : Constant  Value=Lf
  Ra : Gain  Gain=Ra
  Rf : Gain  Gain=Rf
  Sum : Sum  Inputs=|++
  Sum1 : Sum  Inputs=|++
  Sum2 : Sum  Inputs=|+--
  current : Outport
  wires:
  La/1 -> Sum/1
  Divide2/1 -> Sum2/3
  Lf/1 -> Sum/2
  Integrator/1 -> Rf/1, Ra/1, current/1, Laf/1  "i"
  Ra/1 -> Sum1/1
  Rf/1 -> Sum1/2
  omega/1 -> Divide2/2
  Divide1/1 -> Sum2/1
  Sum/1 -> Divide2/3, Divide/2, Divide1/2
  Voltage/1 -> Divide1/1
  Laf/1 -> Divide2/1
  Divide/1 -> Sum2/2
  Sum1/1 -> Divide/1
  Sum2/1 -> Integrator/1  "di/dt"

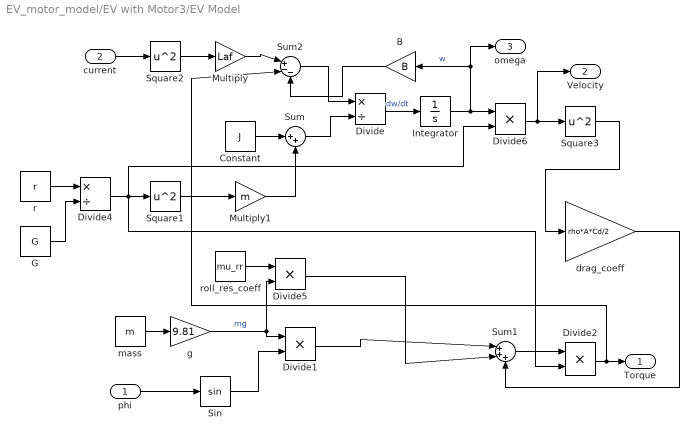
== system EV_motor_model/EV with Motor3/EV Model ==
  phi : Inport
  current : Inport  Port=2
  B : Gain  Gain=B
  Constant : Constant  Value=J
  Divide : Product  Inputs=*/
  Divide{1..2,5..6} (4 alike) : Product  Inputs=**
  Divide4 : Product  Inputs=*/
  G : Constant  Value=G
  Integrator : Integrator
  Multiply : Gain  Gain=Laf
  Multiply1 : Gain  Gain=m
  Sin : Trigonometry
  Square1 : Math  Operator=square
  Square2 : Math  Operator=square
  Square3 : Math  Operator=square
  Sum : Sum  Inputs=|++
  Sum1 : Sum  Inputs=|+++
  Sum2 : Sum  Inputs=|+--
  drag_coeff : Gain  Gain=rho*A*Cd/2
  g : Gain  Gain=9.81
  mass : Constant  Value=m
  r : Constant  Value=r
  roll_res_coeff : Constant  Value=mu_rr
  Torque : Outport
  Velocity : Outport  Port=2
  omega : Outport  Port=3
  wires:
  Sum/1 -> Divide/2
  Divide6/1 -> Velocity/1, Square3/1
  g/1 -> Divide5/2, Divide1/1  "mg"
  current/1 -> Square2/1
  B/1 -> Sum2/3
  Constant/1 -> Sum/1
  Multiply1/1 -> Sum/2
  r/1 -> Divide4/1
  Sum1/1 -> Divide2/1
  Square1/1 -> Multiply1/1
  Sum2/1 -> Divide/1
  Integrator/1 -> Divide6/1, omega/1, B/1  "w"
  phi/1 -> Sin/1
  roll_res_coeff/1 -> Divide5/1
  Multiply/1 -> Sum2/1
  Divide1/1 -> Sum1/1
  Square2/1 -> Multiply/1
  Divide5/1 -> Sum1/2
  mass/1 -> g/1
  Square3/1 -> drag_coeff/1
  G/1 -> Divide4/2
  Divide/1 -> Integrator/1  "dw/dt"
  Divide4/1 -> Divide6/2, Divide2/2, Square1/1
  drag_coeff/1 -> Sum1/3
  Divide2/1 -> Sum2/2, Torque/1
  Sin/1 -> Divide1/2
